simulink model "acm_robot_model_2017b_final"  (R2020a)
settings: Solver=ode4  StartTime=0.0  StopTime=30  FixedStep=1e-3  RelTol=1e-3
InitFcn:
  | acm_init
values from neighbouring files (symbols this model uses):
  alpha = 10*eye(2)    [acm_init.m]    (also in acm_init_final.m; calculating_YQ.m = 1)
  beta = 1    [acm_init.m]    (also in acm_init_final.m)
  fd1 = 5.3    [acm_init.m]    (also in acm_init_final.m; calculating_YQ.m)
  fd2 = 1.1    [acm_init.m]    (also in acm_init_final.m; calculating_YQ.m)
  gamma = 2*eye(5)    [acm_init.m]    (also in acm_init_final.m = 10*eye(5))
  K = 10*eye(2)    [acm_init.m]    (also in acm_init_final.m = 100*eye(2))
  p1 = 3.473    [acm_init.m]    (also in acm_init_final.m; calculating_YQ.m)
  p2 = 0.196    [acm_init.m]    (also in acm_init_final.m; calculating_YQ.m)
  p3 = 0.242    [acm_init.m]    (also in acm_init_final.m; calculating_YQ.m)
settings Model: Creator=Tenghu  LastModifiedBy=User
settings SolverCC: ZeroCrossControl=EnableAll  AlgebraicLoopSolver=LineSearch
settings DataIOCC: SaveFormat=StructureWithTime
settings OptimizationCC: BlockReduction=off  BooleanDataType=off  LifeSpan=inf
settings DebuggingCC: SaveWithParameterizedLinksMsg=none  UnderspecifiedInitializationDetection=Classic  MergeDetectMultiDrivingBlocksExec=none  SignalResolutionControl=TryResolveAllWithWarning  AllowSymbolicDim=off  SFUnexpectedBacktrackingDiag=warning  SFNoUnconditionalDefaultTransitionDiag=warning  SFExecutionAtInitializationDiag=none  ArithmeticOperatorsInVariantConditions=warning
settings HardwareCC: ProdBitPerPointer=32  ProdBitPerSizeT=32  ProdBitPerPtrDiffT=32  ProdLargestAtomicFloat=None  ProdIntDivRoundTo=Undefined  ProdEndianess=Unspecified  ProdWordSize=32  ProdHWDeviceType=32-bit Generic  TargetBitPerPointer=64  TargetBitPerSizeT=64  TargetBitPerPtrDiffT=64  TargetLongLongMode=on  TargetIntDivRoundTo=Zero  TargetEndianess=LittleEndian  TargetWordSize=64  TargetHWDeviceType=MATLAB Host  ProdEqTarget=off
settings ModelReferenceCC: PropagateSignalLabelsOutOfModel=off
settings SFSimCC: SimUseLocalCustomCode=off  CustomCodeUndefinedFunction=UseInterfaceOnly
settings RTWCC: RTWUseLocalCustomCode=off
settings CodeAppCC: StateflowObjectComments=on
settings GRTTargetCC: TargetLangStandard=C89/C90 (ANSI)
settings ConfigComp: CovMetricSettings=dw  CovHtmlReporting=on  CovSaveCumulativeToWorkspaceVar=on  CovSaveSingleToWorkspaceVar=on  CovExternalEMLEnable=off  CovSFcnEnable=off

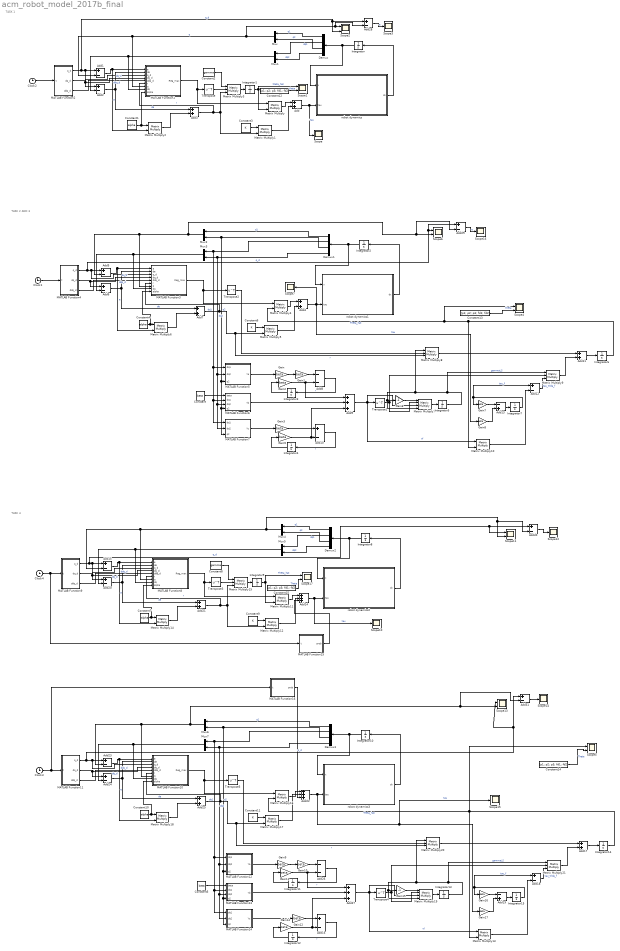
== system acm_robot_model_2017b_final ==
  note: TASK 1
  note: TASK 2 AND 3
  note: TASK 4
  Add{,3..4,7,11,17,21,25} (8 alike) : Sum
  Add{1..2,5..6,10,12,15..16,18,20,23..24,28..31} (16 alike) : Sum  Inputs=+-
  Add13 : Sum  Inputs=-+
  Add{9,14,22,27} (4 alike) : Sum  Inputs=+++
  Add19 : Sum  Inputs=-+
  Add26 : Sum  Inputs=--
  Add8 : Sum  Inputs=--
  Clock{1..4} (4 alike) : Clock
  Constant : Constant  Value=beta
  Constant{1,4,7,10} (4 alike) : Constant  Value=alpha
  Constant{3,6,9,11} (4 alike) : Constant  Value=K
  Constant{12..15} (4 alike) : Constant  Value=[p1; p2; p3; fd1; fd2]
  Constant2 : Constant  Value=gamma
  Constant5 : Constant  Value=beta
  Constant8 : Constant  Value=gamma
  Demux{,1..3} (4 alike) : Demux
  Gain{,1..3,5,7..12,14,16..17} (14 alike) : Gain  Gain=beta
  Gain15 : Gain  Gain=-1
  Gain6 : Gain  Gain=-1
  Integrator{,2,8,10} (4 alike) : Integrator  InitialCondition=[0;0;0;0]
  Integrator{1,3..4,6..7,9,11..12,14..15} (10 alike) : Integrator
  Integrator13 : Integrator  InitialCondition=[1 0 0 0 0; 0 1 0 0 0; 0 0 1 0 0; 0 0 0 1 0; 0 0 0 0 1]
  Integrator5 : Integrator  InitialCondition=[1 0 0 0 0; 0 1 0 0 0; 0 0 1 0 0; 0 0 0 1 0; 0 0 0 0 1]
  MATLAB Function1 : MATLAB Function  TreatAsAtomicUnit=on
  MATLAB Function10 : MATLAB Function  TreatAsAtomicUnit=on
  MATLAB Function11 : MATLAB Function  TreatAsAtomicUnit=on
  MATLAB Function12 : MATLAB Function  TreatAsAtomicUnit=on
  MATLAB Function13 : MATLAB Function  TreatAsAtomicUnit=on
  MATLAB Function14 : MATLAB Function  TreatAsAtomicUnit=on
  MATLAB Function15 : MATLAB Function  TreatAsAtomicUnit=on
  MATLAB Function16 : MATLAB Function  TreatAsAtomicUnit=on
  MATLAB Function2 : MATLAB Function  TreatAsAtomicUnit=on
  MATLAB Function3 : MATLAB Function  TreatAsAtomicUnit=on
  MATLAB Function4 : MATLAB Function  TreatAsAtomicUnit=on
  MATLAB Function5 : MATLAB Function  TreatAsAtomicUnit=on
  MATLAB Function6 : MATLAB Function  TreatAsAtomicUnit=on
  MATLAB Function7 : MATLAB Function  TreatAsAtomicUnit=on
  MATLAB Function8 : MATLAB Function  TreatAsAtomicUnit=on
  MATLAB Function9 : MATLAB Function  TreatAsAtomicUnit=on
  Matrix Multiply{,1..2,4..6,10..14,16..18} (14 alike) : Product  Multiplication=Matrix(*)
  Matrix Multiply{3,8..9,15,20..21} (6 alike) : Product  Inputs=3  Multiplication=Matrix(*)
  Matrix Multiply19 : Product  Inputs=4  Multiplication=Matrix(*)
  Matrix Multiply7 : Product  Inputs=4  Multiplication=Matrix(*)
  Mux{,1..7} (8 alike) : Mux  Inputs=2
  Scope{,3,7,10,12,14..16} (8 alike) : Scope
  Scope{1..2,4..6,11,13,17} (8 alike) : Scope  NumInputPorts=2
  Transpose{,1..5} (6 alike) : Math  Operator=transpose  SaturateOnIntegerOverflow=on
  robot dynamics : MATLAB Function  TreatAsAtomicUnit=on
  robot dynamics1 : MATLAB Function  TreatAsAtomicUnit=on
  robot dynamics2 : MATLAB Function  TreatAsAtomicUnit=on
  robot dynamics3 : MATLAB Function  TreatAsAtomicUnit=on
  wires:
  Clock2/1 -> MATLAB Function2/1(t)
  Add/1 -> Scope/1, robot dynamics/2(tau)  "tau"
  MATLAB Function1/1(Reg_max) -> Transpose/1, Matrix Multiply/1
  Matrix Multiply/1 -> Add/1
  Matrix Multiply1/1 -> Add/2
  Add3/1 -> Matrix Multiply1/2, Matrix Multiply3/3, MATLAB Function1/6(r)  "r"
  MATLAB Function2/1(q_d) -> Add28/1, Scope2/2, MATLAB Function1/3(q_d), Add1/1  "q_d"
  MATLAB Function2/2(dq_d) -> Add2/1, MATLAB Function1/4(dq_d)  "dq_d"
  Add1/1 -> Matrix Multiply2/2, MATLAB Function1/1(e)  "e"
  Add2/1 -> MATLAB Function1/2(de), Add3/1  "de"
  MATLAB Function2/3(ddq_d) -> MATLAB Function1/5(ddq_d)  "ddq_d"
  Constant1/1 -> MATLAB Function1/9(alpha), Matrix Multiply2/1
  Matrix Multiply2/1 -> Add3/2
  Demux/1 -> Mux/1  "q1"
  Demux/3 -> Mux/2  "q2"
  Integrator/1 -> robot dynamics/1(x), Demux/1
  robot dynamics/1(dx) -> Integrator/1
  Demux/2 -> Mux1/1  "dq1"
  Demux/4 -> Mux1/2  "dq2"
  Mux/1 -> Add28/2, Scope2/1, MATLAB Function1/7(q), Add1/2  "q"
  Mux1/1 -> MATLAB Function1/8(dq), Add2/2
  Transpose/1 -> Matrix Multiply3/2
  Constant2/1 -> Matrix Multiply3/1
  Matrix Multiply3/1 -> Integrator1/1
  Integrator1/1 -> Matrix Multiply/2, Scope1/1  "theta_hat"
  Constant3/1 -> Matrix Multiply1/1
  Demux1/2 -> MATLAB Function7/1(dq1), MATLAB Function6/2(dq1), MATLAB Function5/1(dq1), Mux3/1  "dq1"
  Demux1/1 -> Mux2/1  "q1"
  robot dynamics1/1(dx) -> Integrator2/1
  Matrix Multiply4/1 -> Add4/1
  Matrix Multiply6/1 -> Add7/2
  Add7/1 -> Matrix Multiply8/3, Matrix Multiply5/2, MATLAB Function3/6(r)  "r"
  Clock1/1 -> MATLAB Function4/1(t)
  Matrix Multiply5/1 -> Add4/2
  MATLAB Function3/1(Reg_max) -> Transpose2/1, Matrix Multiply4/1
  MATLAB Function4/3(ddq_d) -> MATLAB Function3/5(ddq_d)  "ddq_d"
  Add4/1 -> Scope7/1, Gain8/1, robot dynamics1/2(tau)  "tau"
  Constant6/1 -> Matrix Multiply5/1
  MATLAB Function4/1(q_d) -> Add29/1, Scope6/1, MATLAB Function3/3(q_d), Add5/1  "q_d"
  Integrator2/1 -> robot dynamics1/1(x), Demux1/1
  Mux3/1 -> MATLAB Function3/8(dq), Add6/2
  Demux1/4 -> MATLAB Function7/2(dq2), MATLAB Function6/3(dq2), MATLAB Function5/2(dq2), Mux3/2  "dq2"
  Add6/1 -> MATLAB Function3/2(de), Add7/1  "de"
  Demux1/3 -> MATLAB Function7/3(q2), MATLAB Function6/4(q2), MATLAB Function5/3(q2), Mux2/2  "q2"
  Mux2/1 -> Add29/2, Scope6/2, MATLAB Function3/7(q), Add5/2
  MATLAB Function4/2(dq_d) -> Add6/1, MATLAB Function3/4(dq_d)  "dq_d"
  Add5/1 -> Matrix Multiply6/2, MATLAB Function3/1(e)  "e"
  Constant4/1 -> MATLAB Function3/9(alpha), Matrix Multiply6/1
  Constant/1 -> MATLAB Function6/1(beta)
  MATLAB Function5/1(Ya) -> Gain/1
  Gain/1 -> Gain1/1
  Gain1/1 -> Add8/1
  Add8/1 -> Integrator3/1  "r"
  Integrator3/1 -> Gain2/1
  Gain2/1 -> Add9/1, Add8/2
  MATLAB Function6/1(Yb) -> Add9/2
  Gain5/1 -> Add9/3, Add10/2
  Integrator4/1 -> Gain5/1
  Add10/1 -> Integrator4/1  "r"
  Gain3/1 -> Add10/1
  MATLAB Function7/1(Yc) -> Gain3/1
  Add9/1 -> Matrix Multiply10/1, Matrix Multiply7/3, Transpose1/1  "Yf"
  Matrix Multiply7/1 -> Integrator5/1
  Transpose1/1 -> Matrix Multiply9/2, Matrix Multiply7/2
  Integrator5/1 -> Matrix Multiply9/1, Matrix Multiply8/1, Matrix Multiply7/4, Gain6/1  "gammaLS"
  Gain6/1 -> Matrix Multiply7/1
  Transpose2/1 -> Matrix Multiply8/2
  Matrix Multiply8/1 -> Add11/1
  Matrix Multiply9/1 -> Add11/2
  Add11/1 -> Integrator6/1
  Integrator6/1 -> Matrix Multiply10/2, Scope4/1, Matrix Multiply4/2  "Theta_hat"
  Add12/1 -> Matrix Multiply9/3  "tau_tilda_f"
  Matrix Multiply10/1 -> Add12/2
  Integrator7/1 -> Add12/1, Gain7/1  "tau_f"
  Add13/1 -> Integrator7/1
  Gain7/1 -> Add13/1
  Gain8/1 -> Add13/2
  MATLAB Function11/2(dq_d) -> Add24/1, MATLAB Function10/4(dq_d)  "dq_d"
  Transpose3/1 -> Matrix Multiply15/2
  Gain12/1 -> Add16/1
  Demux3/3 -> MATLAB Function14/3(q2), MATLAB Function13/4(q2), MATLAB Function12/3(q2), Mux6/2  "q2"
  Integrator10/1 -> robot dynamics3/1(x), Demux3/1
  Add22/1 -> Scope15/1, Gain17/1, robot dynamics3/2(tau)  "tau"
  Matrix Multiply12/1 -> Add14/2
  Matrix Multiply16/1 -> Add22/1
  MATLAB Function8/1(Reg_max) -> Transpose3/1, Matrix Multiply11/1
  MATLAB Function9/3(ddq_d) -> MATLAB Function8/5(ddq_d)  "ddq_d"
  Constant5/1 -> MATLAB Function13/1(beta)
  Demux3/4 -> MATLAB Function14/2(dq2), MATLAB Function13/3(dq2), MATLAB Function12/2(dq2), Mux7/2  "dq2"
  MATLAB Function9/1(q_d) -> Scope11/1, Add30/1, MATLAB Function8/3(q_d), Add15/1  "q_d"
  Constant11/1 -> Matrix Multiply17/1
  Matrix Multiply14/1 -> Add21/2
  Matrix Multiply11/1 -> Add14/1
  Add19/1 -> Integrator15/1
  Matrix Multiply15/1 -> Integrator9/1
  Constant9/1 -> Matrix Multiply12/1
  Demux2/4 -> Mux5/2  "dq2"
  Matrix Multiply19/1 -> Integrator13/1
  Gain17/1 -> Add19/2
  Clock4/1 -> MATLAB Function15/1(t), MATLAB Function9/1(t)
  Add20/1 -> MATLAB Function8/2(de), Add21/1  "de"
  robot dynamics3/1(dx) -> Integrator10/1
  Demux2/3 -> Mux4/2  "q2"
  Mux4/1 -> Add30/2, Scope11/2, MATLAB Function8/7(q), Add15/2
  Mux5/1 -> MATLAB Function8/8(dq), Add20/2
  Demux2/1 -> Mux4/1  "q1"
  Add25/1 -> Matrix Multiply20/3, Matrix Multiply17/2, MATLAB Function10/6(r)  "r"
  Add21/1 -> Matrix Multiply12/2, Matrix Multiply15/3, MATLAB Function8/6(r)  "r"
  Add24/1 -> MATLAB Function10/2(de), Add25/1  "de"
  robot dynamics2/1(dx) -> Integrator8/1
  MATLAB Function9/2(dq_d) -> Add20/1, MATLAB Function8/4(dq_d)  "dq_d"
  Add14/1 -> Scope10/1, robot dynamics2/2(tau)  "tau"
  MATLAB Function10/1(Reg_max) -> Transpose5/1, Matrix Multiply16/1
  Add15/1 -> Matrix Multiply14/2, MATLAB Function8/1(e)  "e"
  MATLAB Function11/1(q_d) -> Scope13/1, Add31/1, MATLAB Function10/3(q_d), Add23/1  "q_d"
  Integrator12/1 -> Gain14/1
  Integrator15/1 -> Add18/1, Gain16/1  "tau_f"
  Constant7/1 -> MATLAB Function8/9(alpha), Matrix Multiply14/1
  Transpose4/1 -> Matrix Multiply21/2, Matrix Multiply19/2
  Constant8/1 -> Matrix Multiply15/1
  Integrator13/1 -> Matrix Multiply21/1, Matrix Multiply20/1, Matrix Multiply19/4, Gain15/1  "gammaLS"
  MATLAB Function11/3(ddq_d) -> MATLAB Function10/5(ddq_d)  "ddq_d"
  Add17/1 -> Integrator14/1
  Add26/1 -> Integrator11/1  "r"
  Matrix Multiply17/1 -> Add22/2
  Demux3/1 -> Mux6/1  "q1"
  Add27/1 -> Matrix Multiply13/1, Matrix Multiply19/3, Transpose4/1  "Yf"
  Matrix Multiply18/1 -> Add25/2
  Integrator8/1 -> robot dynamics2/1(x), Demux2/1
  Constant10/1 -> MATLAB Function10/9(alpha), Matrix Multiply18/1
  Demux2/2 -> Mux5/1  "dq1"
  Clock3/1 -> MATLAB Function16/1(t), MATLAB Function11/1(t)
  Mux7/1 -> MATLAB Function10/8(dq), Add24/2
  Mux6/1 -> Add31/2, Scope13/2, MATLAB Function10/7(q), Add23/2
  Add23/1 -> Matrix Multiply18/2, MATLAB Function10/1(e)  "e"
  Add18/1 -> Matrix Multiply21/3  "tau_tilda_f"
  Gain14/1 -> Add27/3, Add16/2
  Demux3/2 -> MATLAB Function14/1(dq1), MATLAB Function13/2(dq1), MATLAB Function12/1(dq1), Mux7/1  "dq1"
  Matrix Multiply20/1 -> Add17/1
  MATLAB Function14/1(Yc) -> Gain12/1
  Matrix Multiply13/1 -> Add18/2
  Matrix Multiply21/1 -> Add17/2
  MATLAB Function13/1(Yb) -> Add27/2
  Gain11/1 -> Add27/1, Add26/2
  Integrator11/1 -> Gain11/1
  Add16/1 -> Integrator12/1  "r"
  Gain16/1 -> Add19/1
  Transpose5/1 -> Matrix Multiply20/2
  Gain15/1 -> Matrix Multiply19/1
  Gain9/1 -> Gain10/1
  Gain10/1 -> Add26/1
  MATLAB Function12/1(Ya) -> Gain9/1
  MATLAB Function15/1(prob) -> Add14/3
  MATLAB Function16/1(prob) -> Add22/3
  Constant12/1 -> Scope1/2  "theta"
  Add28/1 -> Scope3/1  "e"
  Constant13/1 -> Scope4/2  "theta"
  Add29/1 -> Scope16/1  "e"
  Integrator14/1 -> Scope5/1, Matrix Multiply13/2, Matrix Multiply16/2  "Theta_hat"
  Constant14/1 -> Scope5/2  "Theta"
  Constant15/1 -> Scope17/2  "Theta"
  Integrator9/1 -> Scope17/1, Matrix Multiply11/2  "Theta_hat"
  Add30/1 -> Scope12/1
  Add31/1 -> Scope14/1

== matlab function acm_robot_model_2017b_final/MATLAB Function2 ==
  data: t input; q_d output; dq_d output; ddq_d output
function [q_d, dq_d, ddq_d]  = desired_traj(t)
    q_d = [sin(3*t);2*cos(t)];
    dq_d = [3*cos(3*t);-2*sin(t)];
    ddq_d = [-9*sin(3*t);-2*cos(t)];
end

== matlab function acm_robot_model_2017b_final/MATLAB Function7 ==
  data: dq1 input; Yc output; dq2 input; q2 input
function Yc = Yc(dq1,dq2,q2)

Yc = [0,0,0,dq1,0; 0, 0, sin(q2)*(dq1*dq2+dq1^2), 0, dq2];
end

== matlab function acm_robot_model_2017b_final/MATLAB Function10 ==
  data: e input; Reg_max output; de input; q_d input; dq_d input; ddq_d input; r input; q input; dq input; alpha input
function Reg_max   = Y(e, de, q_d, dq_d, ddq_d, r, q, dq, alpha)
    alpha=alpha(1,1);
    Q=[ddq_d(1)+alpha*de(1),ddq_d(2)+alpha*de(2);
        dq_d(1)+alpha*e(1),dq_d(2)+alpha*e(2);
        dq_d(1)+alpha*e(1)-r(1),dq_d(2)+alpha*e(2)-r(2)];
    Reg_max=[Q(1,1),  Q(1,2),  2*cos(q(2))*Q(1,1)+cos(q(2))*Q(1,2)-sin(q(2))*dq(2)*Q(2,1)-sin(q(2))*(dq(1)+dq(2))*Q(2,2),  Q(3,1),  0;
             0,  Q(1,1)+Q(1,2),  cos(q(2))*Q(1,1)+sin(q(2))*dq(1)*Q(2,1),0 , Q(3,2)];
end

== matlab function acm_robot_model_2017b_final/MATLAB Function11 ==
  data: t input; q_d output; dq_d output; ddq_d output
function [q_d, dq_d, ddq_d]  = desired_traj(t)
    q_d = [sin(3*t);2*cos(t)];
    dq_d = [3*cos(3*t);-2*sin(t)];
    ddq_d = [-9*sin(3*t);-2*cos(t)];
end

== matlab function acm_robot_model_2017b_final/MATLAB Function12 ==
  data: dq1 input; Ya output; dq2 input; q2 input
function Ya = Ya(dq1,dq2,q2)

Ya = [dq1,dq2,cos(q2)*(dq1*2+dq2),0,0; 0.0,dq1+dq2,dq1*cos(q2),0,0];

== matlab function acm_robot_model_2017b_final/MATLAB Function13 ==
  data: beta input; Yb output; dq1 input; dq2 input; q2 input
function Yb = Yb(beta,dq1,dq2,q2)

Yb = [beta*dq1,beta*dq2,beta*cos(q2)*(dq1*2+dq2),0,0; 0, beta*(dq1+dq2), beta*dq1*cos(q2),0 ,0];
end

== matlab function acm_robot_model_2017b_final/MATLAB Function14 ==
  data: dq1 input; Yc output; dq2 input; q2 input
function Yc = Yc(dq1,dq2,q2)

Yc = [0,0,0,dq1,0; 0, 0, sin(q2)*(dq1*dq2+dq1^2), 0, dq2];
end

== matlab function acm_robot_model_2017b_final/MATLAB Function8 ==
  data: e input; Reg_max output; de input; q_d input; dq_d input; ddq_d input; r input; q input; dq input; alpha input
function Reg_max   = Y(e, de, q_d, dq_d, ddq_d, r, q, dq, alpha)
    alpha=alpha(1,1);
    Q=[ddq_d(1)+alpha*de(1),ddq_d(2)+alpha*de(2);
        dq_d(1)+alpha*e(1),dq_d(2)+alpha*e(2);
        dq_d(1)+alpha*e(1)-r(1),dq_d(2)+alpha*e(2)-r(2)];
    Reg_max=[Q(1,1),  Q(1,2),  2*cos(q(2))*Q(1,1)+cos(q(2))*Q(1,2)-sin(q(2))*dq(2)*Q(2,1)-sin(q(2))*(dq(1)+dq(2))*Q(2,2),  Q(3,1),  0;
             0,  Q(1,1)+Q(1,2),  cos(q(2))*Q(1,1)+sin(q(2))*dq(1)*Q(2,1),0 , Q(3,2)];
end

== matlab function acm_robot_model_2017b_final/MATLAB Function9 ==
  data: t input; q_d output; dq_d output; ddq_d output
function [q_d, dq_d, ddq_d]  = desired_traj(t)
    q_d = [sin(3*t);2*cos(t)];
    dq_d = [3*cos(3*t);-2*sin(t)];
    ddq_d = [-9*sin(3*t);-2*cos(t)];
end

== matlab function acm_robot_model_2017b_final/robot dynamics2 ==
  data: x input; dx output; tau input; p1 parameter; p2 parameter; p3 parameter; fd1 parameter; fd2 parameter
% *************************************************************************
%                        2-Link Manipulator Dynamics                      *
% *************************************************************************

function dx = fcn_twoLinkDynamics(x, tau, p1, p2, p3, fd1, fd2)
    q1  = x(1);
    dq1 = x(2);
    q2  = x(3);
    dq2 = x(4);
    
    M      = zeros(2,2);
    M(1,1) = p1 + 2*p3*cos(q2);
    M(1,2) = p2 + p3*cos(q2);
    M(2,1) = p2 + p3*cos(q2);
    M(2,2) = p2;

    C      = zeros(2,2);
    C(1,1) = -p3*sin(q2)*dq2;
    C(1,2) = -p3*sin(q2)*(dq1+dq2);
    C(2,1) = p3*sin(q2)*dq1;
    C(2,2) = 0;

    Fd     = diag([fd1 fd2]);

    % The system without bounded disturbances =============================
    ddq = M\(tau - C*[dq1;dq2] - Fd*[dq1;dq2]);
    dx  = [dq1; ddq(1); dq2; ddq(2)];
end

== matlab function acm_robot_model_2017b_final/MATLAB Function1 ==
  data: e input; Reg_max output; de input; q_d input; dq_d input; ddq_d input; r input; q input; dq input; alpha input
function Reg_max   = Y(e, de, q_d, dq_d, ddq_d, r, q, dq, alpha)
    alpha=alpha(1,1);
    Q=[ddq_d(1)+alpha*de(1),ddq_d(2)+alpha*de(2);
        dq_d(1)+alpha*e(1),dq_d(2)+alpha*e(2);
        dq_d(1)+alpha*e(1)-r(1),dq_d(2)+alpha*e(2)-r(2)];
    Reg_max=[Q(1,1),  Q(1,2),  2*cos(q(2))*Q(1,1)+cos(q(2))*Q(1,2)-sin(q(2))*dq(2)*Q(2,1)-sin(q(2))*(dq(1)+dq(2))*Q(2,2),  Q(3,1),  0;
             0,  Q(1,1)+Q(1,2),  cos(q(2))*Q(1,1)+sin(q(2))*dq(1)*Q(2,1),0 , Q(3,2)];
end

== matlab function acm_robot_model_2017b_final/robot dynamics3 ==
  data: x input; dx output; tau input; p1 parameter; p2 parameter; p3 parameter; fd1 parameter; fd2 parameter
% *************************************************************************
%                        2-Link Manipulator Dynamics                      *
% *************************************************************************

function dx = fcn_twoLinkDynamics(x, tau, p1, p2, p3, fd1, fd2)
    q1  = x(1);
    dq1 = x(2);
    q2  = x(3);
    dq2 = x(4);
    
    M      = zeros(2,2);
    M(1,1) = p1 + 2*p3*cos(q2);
    M(1,2) = p2 + p3*cos(q2);
    M(2,1) = p2 + p3*cos(q2);
    M(2,2) = p2;

    C      = zeros(2,2);
    C(1,1) = -p3*sin(q2)*dq2;
    C(1,2) = -p3*sin(q2)*(dq1+dq2);
    C(2,1) = p3*sin(q2)*dq1;
    C(2,2) = 0;

    Fd     = diag([fd1 fd2]);

    % The system without bounded disturbances =============================
    ddq = M\(tau - C*[dq1;dq2] - Fd*[dq1;dq2]);
    dx  = [dq1; ddq(1); dq2; ddq(2)];
end

== matlab function acm_robot_model_2017b_final/MATLAB Function15 ==
  data: t input; prob output
function prob  = prob(t)
    prob = [exp(-0.05*t)*tanh(10*t)*(-10*sin(7*pi*t)+5*sin(exp(t))); exp(-0.05*t)*tanh(10*t)*(-10*sin(9*pi*t) + 10*sin(exp(2*t)))];
end

== matlab function acm_robot_model_2017b_final/MATLAB Function16 ==
  data: t input; prob output
function prob  = prob(t)
    prob = [exp(-0.05*t)*tanh(10*t)*(-10*sin(7*pi*t)+5*sin(exp(t))); exp(-0.05*t)*tanh(10*t)*(-10*sin(9*pi*t) + 10*sin(exp(2*t)))];
end

== matlab function acm_robot_model_2017b_final/MATLAB Function3 ==
  data: e input; Reg_max output; de input; q_d input; dq_d input; ddq_d input; r input; q input; dq input; alpha input
function Reg_max   = Y(e, de, q_d, dq_d, ddq_d, r, q, dq, alpha)
    alpha=alpha(1,1);
    Q=[ddq_d(1)+alpha*de(1),ddq_d(2)+alpha*de(2);
        dq_d(1)+alpha*e(1),dq_d(2)+alpha*e(2);
        dq_d(1)+alpha*e(1)-r(1),dq_d(2)+alpha*e(2)-r(2)];
    Reg_max=[Q(1,1),  Q(1,2),  2*cos(q(2))*Q(1,1)+cos(q(2))*Q(1,2)-sin(q(2))*dq(2)*Q(2,1)-sin(q(2))*(dq(1)+dq(2))*Q(2,2),  Q(3,1),  0;
             0,  Q(1,1)+Q(1,2),  cos(q(2))*Q(1,1)+sin(q(2))*dq(1)*Q(2,1),0 , Q(3,2)];
end

== matlab function acm_robot_model_2017b_final/MATLAB Function4 ==
  data: t input; q_d output; dq_d output; ddq_d output
function [q_d, dq_d, ddq_d]  = desired_traj(t)
    q_d = [sin(3*t);2*cos(t)];
    dq_d = [3*cos(3*t);-2*sin(t)];
    ddq_d = [-9*sin(3*t);-2*cos(t)];
end

== matlab function acm_robot_model_2017b_final/robot dynamics ==
  data: x input; dx output; tau input; p1 parameter; p2 parameter; p3 parameter; fd1 parameter; fd2 parameter
% *************************************************************************
%                        2-Link Manipulator Dynamics                      *
% *************************************************************************

function dx = fcn_twoLinkDynamics(x, tau, p1, p2, p3, fd1, fd2)
    q1  = x(1);
    dq1 = x(2);
    q2  = x(3);
    dq2 = x(4);
    
    M      = zeros(2,2);
    M(1,1) = p1 + 2*p3*cos(q2);
    M(1,2) = p2 + p3*cos(q2);
    M(2,1) = p2 + p3*cos(q2);
    M(2,2) = p2;

    C      = zeros(2,2);
    C(1,1) = -p3*sin(q2)*dq2;
    C(1,2) = -p3*sin(q2)*(dq1+dq2);
    C(2,1) = p3*sin(q2)*dq1;
    C(2,2) = 0;

    Fd     = diag([fd1 fd2]);

    % The system without bounded disturbances =============================
    ddq = M\(tau - C*[dq1;dq2] - Fd*[dq1;dq2]);
    dx  = [dq1; ddq(1); dq2; ddq(2)];
end

== matlab function acm_robot_model_2017b_final/robot dynamics1 ==
  data: x input; dx output; tau input; p1 parameter; p2 parameter; p3 parameter; fd1 parameter; fd2 parameter
% *************************************************************************
%                        2-Link Manipulator Dynamics                      *
% *************************************************************************

function dx = fcn_twoLinkDynamics(x, tau, p1, p2, p3, fd1, fd2)
    q1  = x(1);
    dq1 = x(2);
    q2  = x(3);
    dq2 = x(4);
    
    M      = zeros(2,2);
    M(1,1) = p1 + 2*p3*cos(q2);
    M(1,2) = p2 + p3*cos(q2);
    M(2,1) = p2 + p3*cos(q2);
    M(2,2) = p2;

    C      = zeros(2,2);
    C(1,1) = -p3*sin(q2)*dq2;
    C(1,2) = -p3*sin(q2)*(dq1+dq2);
    C(2,1) = p3*sin(q2)*dq1;
    C(2,2) = 0;

    Fd     = diag([fd1 fd2]);

    % The system without bounded disturbances =============================
    ddq = M\(tau - C*[dq1;dq2] - Fd*[dq1;dq2]);
    dx  = [dq1; ddq(1); dq2; ddq(2)];
end

== matlab function acm_robot_model_2017b_final/MATLAB Function5 ==
  data: dq1 input; Ya output; dq2 input; q2 input
function Ya = Ya(dq1,dq2,q2)

Ya = [dq1,dq2,cos(q2)*(dq1*2+dq2),0,0; 0.0,dq1+dq2,dq1*cos(q2),0,0];

== matlab function acm_robot_model_2017b_final/MATLAB Function6 ==
  data: beta input; Yb output; dq1 input; dq2 input; q2 input
function Yb = Yb(beta,dq1,dq2,q2)

Yb = [beta*dq1,beta*dq2,beta*cos(q2)*(dq1*2+dq2),0,0; 0, beta*(dq1+dq2), beta*dq1*cos(q2),0 ,0];
end
